simulink model "add_entry_model_tester_3"  (R2020b)
settings: Solver=FixedStepDiscrete  StartTime=0.0  StopTime=21  FixedStep=0.1  RelTol=1e-3
undefined symbols (not defined in the file or in its folder): DiscIntNeverNeededParam, test_input
libraries: simulink x3
settings Model: Creator=rsub  LastModifiedBy=rsub

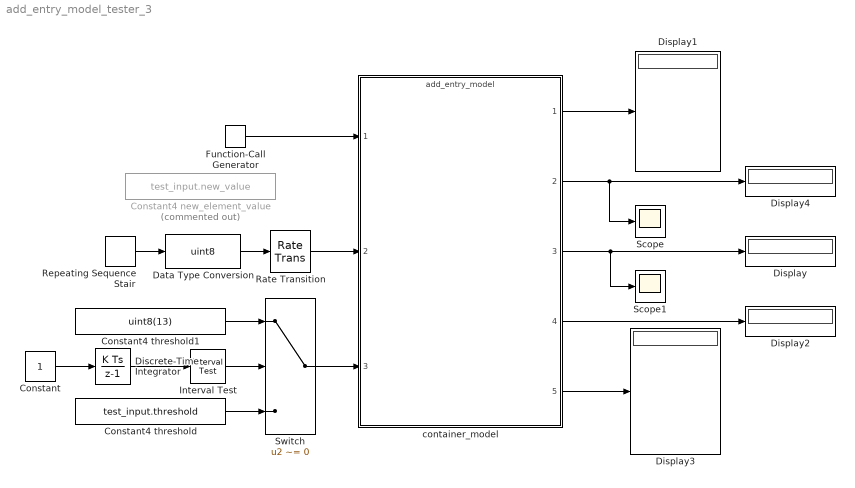
== system add_entry_model_tester_3 ==
  Constant : Constant
  Constant4 new_element_value : Constant  Commented=on  Value=test_input.new_value
  Constant4 threshold : Constant  Value=test_input.threshold
  Constant4 threshold1 : Constant  Value=uint8(13)
  Data Type Conversion : DataTypeConversion  OutDataTypeStr=uint8
  Discrete-Time Integrator : DiscreteIntegrator  SampleTime=-1  ICPrevOutput=DiscIntNeverNeededParam  ICPrevScaledInput=DiscIntNeverNeededParam
  Display{,1..4} (5 alike) : Display
  Function-Call Generator : simulink/Ports & Subsystems/Function-Call Generator  sample_time=5  numberOfIterations=1  DisallowWideOutput=off
  Interval Test : simulink/Logic and Bit Operations/Interval Test  IntervalClosedRight=on  uplimit=19  IntervalClosedLeft=on  lowlimit=14  OutDataTypeStr=boolean
  Rate Transition : RateTransition  Integrity=off  Deterministic=off  OutPortSampleTime=5
  Repeating Sequence Stair : simulink/Sources/Repeating Sequence Stair  OutValues=[10 11 12 13 14 15 15 ].'  tsamp=5  OutMin=[]  OutMax=[]  OutDataTypeStr=double  OutputDataTypeScalingMode=double  OutDataType=fixdt(0,8)  ConRadixGroup=Best Precision: Vector-wise  OutScaling=2^-12
  Scope : Scope
  Scope1 : Scope
  Switch : Switch  Criteria=u2 ~= 0
  container_model : ModelReference  ModelNameDialog=add_entry_model.slx  ScheduleRates=on  ModelReferenceVersion=1.301
  wires:
  container_model/1 -> Display1/1
  container_model/4 -> Display2/1
  container_model/3 -> Scope1/1, Display/1
  container_model/2 -> Scope/1, Display4/1
  Rate Transition/1 -> container_model/2
  container_model/5 -> Display3/1
  Repeating Sequence Stair/1 -> Data Type Conversion/1
  Data Type Conversion/1 -> Rate Transition/1
  Function-Call Generator/1 -> container_model/1
  Constant/1 -> Discrete-Time Integrator/1
  Interval Test/1 -> Switch/2
  Discrete-Time Integrator/1 -> Interval Test/1
  Constant4 threshold/1 -> Switch/3
  Switch/1 -> container_model/3
  Constant4 threshold1/1 -> Switch/1
